simulink model "ControlSystem_Refactorization"  (R2025a)
settings: Solver=FixedStepAuto  StartTime=0.0  StopTime=inf  FixedStep=1e-4  RelTol=1e-3
PostLoadFcn:
  | clear;
  | load_system('ControlSystem_Refactorization');
  | evalin('base', 'run("inicializarBuses.m")');
values from neighbouring files (symbols this model uses):
  actuadorBus = arrayfun(@(x) Simulink.Bus.createMATLABStruct(actuadorBusInfo.busName, x), actuador)    [inicializarBuses.m]
undefined symbols (not defined in the file or in its folder): Configuracion, Controlador, Estado, EstadoValvula, ModoControl, National_Instruments, ParametroControl, PCIe
libraries: simulink x11, sldrtlib x5
(part 1 of 2)
settings Model: SimulationMode=external  ExtModeTrigDuration=10000  Creator=David  LastModifiedBy=David
settings HardwareCC: ProdBitPerLong=64.0  ProdHWDeviceType=Intel->x86-64 (Linux 64)
settings RTWCC: SystemTargetFile=sldrt.tlc  TemplateMakefile=sldrt.tmf  RTWCompilerOptimization=on  Description=Simulink Desktop Real-Time
settings CodeAppCC: MaxIdLength=95.0
settings SimulinkDesktopRealTimeCC: ExtModeTransport=0.0  ExtModeStaticAllocSize=1000000.0  TargetLibSuffix=_sldrt.a  TargetPreCompLibLocation=C:\Program Files\MATLAB\R2025a\toolbox\sldrt\lib\win64  MultiwordLength=2048.0  DynamicStringBufferSize=256.0  ParMdlRefBuildCompliant=on  PreserveMATLABNamespacesInGeneratedCode=on  SubcomponentCodeInterfacePackaging=Reusable function

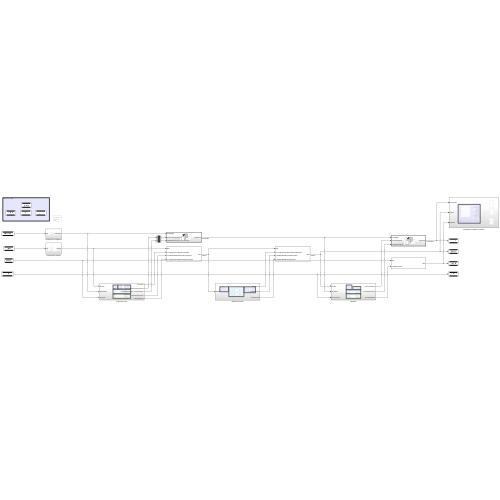
[thumbnail: Simulink's stored preview of the top-level diagram]
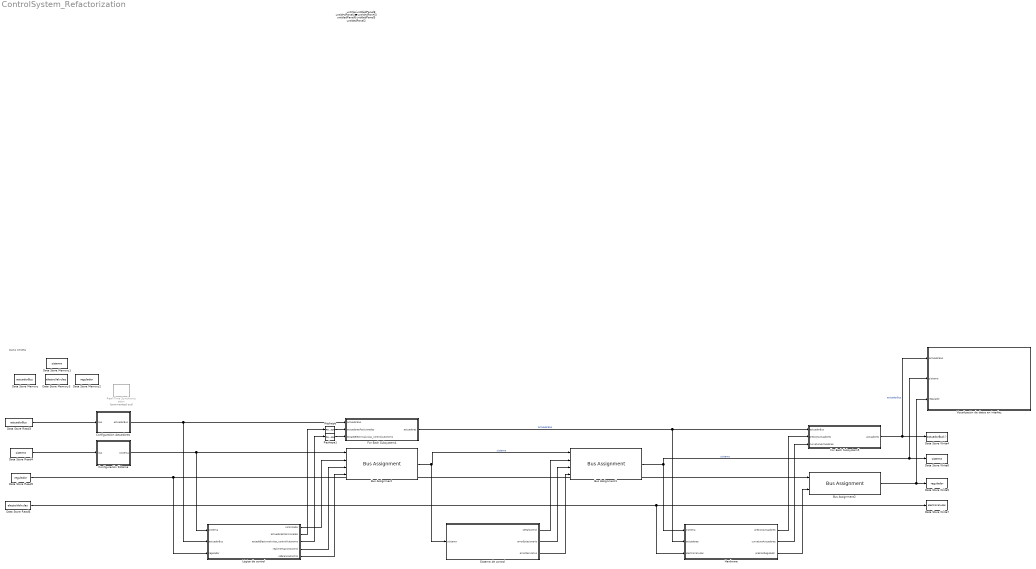
== system ControlSystem_Refactorization ==
  note: DATA STORE
  Bus Assignment : BusAssignment  AssignedSignals=Configuracion.Global.controlador,Estado.Global.realimentacionControl,Configuracion.Global.referenciaControl
  Bus Assignment1 : BusAssignment  AssignedSignals=Configuracion.Global.referenciaControl,Estado.Global.errorEstacionario,Estado.Global.errorDerivativo
  Bus Assignment2 : BusAssignment  AssignedSignals=Estado.presion
  Configuración Actuadores : Subsystem
  Configuración Sistema : Subsystem
  Data Store Memory : DataStoreMemory  DataStoreName=actuadorBus  WriteAfterWriteMsg=warning  InitialValue=actuadorBus  ShowAdditionalParam=off  OutDataTypeStr=Bus: slBusActuador
  Data Store Memory1 : DataStoreMemory  DataStoreName=sistema  WriteAfterWriteMsg=warning  InitialValue=sistema  ShowAdditionalParam=off  OutDataTypeStr=Bus: slBusSistema
  Data Store Memory2 : DataStoreMemory  DataStoreName=regulador  WriteAfterWriteMsg=warning  InitialValue=regulador  ShowAdditionalParam=off  OutDataTypeStr=Bus: slBusRegulador
  Data Store Memory3 : DataStoreMemory  DataStoreName=electroValvulas  WriteAfterWriteMsg=warning  InitialValue=electroValvulas  ShowAdditionalParam=off  OutDataTypeStr=Bus: slBusElectroValvulas
  Data Store Read3 : DataStoreRead  DataStoreName=actuadorBus  IndexOptions=Index vector (dialog)  Indices=1  OutputSizes=1
  Data Store Read4 : DataStoreRead  DataStoreName=sistema  IndexOptions=Index vector (dialog)  Indices=1  OutputSizes=1
  Data Store Read5 : DataStoreRead  DataStoreName=regulador  IndexOptions=Index vector (dialog)  Indices=1  OutputSizes=1
  Data Store Read6 : DataStoreRead  DataStoreName=electroValvulas  IndexOptions=Index vector (dialog)  Indices=1  OutputSizes=1
  Data Store Write4 : DataStoreWrite  DataStoreName=actuadorBus  DataStoreElements=actuadorBus(:)  IndexOptions=Index vector (dialog)  Indices=1  OutputSizes=1
  Data Store Write5 : DataStoreWrite  DataStoreName=regulador  DataStoreElements=regulador  IndexOptions=Index vector (dialog)  Indices=1  OutputSizes=1
  Data Store Write6 : DataStoreWrite  DataStoreName=sistema  DataStoreElements=sistema  IndexOptions=Index vector (dialog)  Indices=1  OutputSizes=1
  Data Store Write7 : DataStoreWrite  DataStoreName=electroValvulas  DataStoreElements=electroValvulas  IndexOptions=Index vector (dialog)  Indices=1  OutputSizes=1
  For Each Subsystem4 : Subsystem  TreatAsAtomicUnit=on
  For Each Subsystem5 : Subsystem  TreatAsAtomicUnit=on
  Hardware : Subsystem
  Lógica de control : Subsystem
  Real-Time Synchronization : sldrtlib/Real-Time Synchronization  Commented=on  SampleTime=0.1  MaxMissedTicks=10  ShowMissedTicks=off  YieldWhenWaiting=off
  Reshape : Reshape  OutputDimensionality=Column vector (2-D)
  Reshape1 : Reshape  OutputDimensionality=Column vector (2-D)
  Sistema de control : Subsystem
  Visualización de datos en interfaz : Subsystem
  untitledPanel : Subsystem  Tag=HiddenForWebPanel  IsWebBlockPanel=on
  untitledPanel1 : Subsystem  Tag=HiddenForWebPanel  IsWebBlockPanel=on
  untitledPanel2 : Subsystem  Tag=HiddenForWebPanel  IsWebBlockPanel=on
  untitledPanel3 : Subsystem  Tag=HiddenForWebPanel  IsWebBlockPanel=on
  untitledPanel4 : Subsystem  Tag=HiddenForWebPanel  IsWebBlockPanel=on
  untitledPanel5 : Subsystem  Tag=HiddenForWebPanel  IsWebBlockPanel=on
  untitledPanel6 : Subsystem  Tag=HiddenForWebPanel  IsWebBlockPanel=on
  untitledPanel8 : Subsystem  Tag=HiddenForWebPanel  IsWebBlockPanel=on
  wires:
  Data Store Read4/1 -> Configuración Sistema/1(bus)
  Data Store Read5/1 -> Lógica de control/3(regulador), Bus Assignment2/1
  Data Store Read3/1 -> Configuración Actuadores/1(bus)
  Lógica de control/1(controlador) -> Bus Assignment/2
  Lógica de control/4(realimentacionControl) -> Bus Assignment/3
  Lógica de control/5(referenciaControl) -> Bus Assignment/4
  Lógica de control/2(actuadoresPosicionados) -> Reshape/1
  Lógica de control/3(estadoElectrovalvulas_controlAutonomo) -> Reshape1/1
  Bus Assignment/1 -> Sistema de control/1(sistema), Bus Assignment1/1  "sistema"
  Sistema de control/1(señalControl) -> Bus Assignment1/2
  Sistema de control/2(errorEstacionario) -> Bus Assignment1/3
  Sistema de control/3(errorDerivativo) -> Bus Assignment1/4
  Bus Assignment1/1 -> Hardware/1(sistema), Visualización de datos en interfaz/2(sistema), Data Store Write6/1  "sistema"
  Data Store Read6/1 -> Data Store Write7/1, Hardware/3(electroValvulas)
  For Each Subsystem4/1(actuadores) -> Hardware/2(actuadores), For Each Subsystem5/1(actuadorBus)  "actuadorBus"
  Hardware/1(presionActuadores) -> For Each Subsystem5/2(presionActuadores)
  Hardware/2(curvaturaActuadores) -> For Each Subsystem5/3(curvaturaActuadores)
  Hardware/3(presiónRegulador) -> Bus Assignment2/2
  For Each Subsystem5/1(actuadores) -> Visualización de datos en interfaz/1(actuadorBus), Data Store Write4/1  "actuadorBus"
  Bus Assignment2/1 -> Visualización de datos en interfaz/3(regulador), Data Store Write5/1
  Reshape/1 -> For Each Subsystem4/2(actuadoresPosicionados)
  Reshape1/1 -> For Each Subsystem4/3(estadoElectrovalvulas_controlAutonomo)
  Configuración Sistema/1(sistema) -> Lógica de control/1(sistema), Bus Assignment/1
  Configuración Actuadores/1(actuadorBus) -> Lógica de control/2(actuadorBus), For Each Subsystem4/1(actuadorBus)

== system ControlSystem_Refactorization/Configuración Actuadores ==
  bus : Inport
  Configuración de usuario : Subsystem  TreatAsAtomicUnit=on
  For Each Subsystem : Subsystem  TreatAsAtomicUnit=on
  actuadorBus : Outport
  wires:
  For Each Subsystem/1(Out1) -> actuadorBus/1
  bus/1 -> For Each Subsystem/1(Bus)
  Configuración de usuario/1(Referencias presión) -> For Each Subsystem/2(Referencias de presión)
  Configuración de usuario/2(Referencias curvatura) -> For Each Subsystem/3(Referencias de curvatura)
  Configuración de usuario/3(Estado válvulas - Control manual) -> For Each Subsystem/4(Estado válvulas - Control manual)
  Configuración de usuario/4(Actuadores activos - Control autónomo) -> For Each Subsystem/5(Actuadores activos - Control autónomo)

== system ControlSystem_Refactorization/Configuración Sistema ==
  bus : Inport
  Bus Assignment3 : BusAssignment  AssignedSignals=Configuracion.Global.modoControl,Configuracion.Global.parametroControl,Configuracion.Global.simulacionActiva,Configuracion.ControlManual.actuadorSeleccionado,Configuracion.Global.ToleranciaPresion.estacionaria,Configuracion.Global.ToleranciaPresion.derivativa,Configuracion.Global.ToleranciaCurvatura.estacionaria,Configuracion.Global.ToleranciaCurvatura.derivativa,Configuracion.Global.toleranciaEquilibrioPresiones
  Configuración de usuario : Subsystem  TreatAsAtomicUnit=on
  sistema : Outport
  wires:
  Bus Assignment3/1 -> sistema/1
  bus/1 -> Bus Assignment3/1
  Configuración de usuario/1(Modo de control) -> Bus Assignment3/2
  Configuración de usuario/2(Parámetro de control) -> Bus Assignment3/3
  Configuración de usuario/3(Simulación activa) -> Bus Assignment3/4
  Configuración de usuario/4(Actuador seleccionado) -> Bus Assignment3/5
  Configuración de usuario/5(Tolerancia Presión Estacionaria) -> Bus Assignment3/6
  Configuración de usuario/6(Tolerancia Presión Derivativa) -> Bus Assignment3/7
  Configuración de usuario/7(Tolerancia Curvatura Estacionaria) -> Bus Assignment3/8
  Configuración de usuario/8(Tolerancia Curvatura Derivativa) -> Bus Assignment3/9
  Configuración de usuario/9(Tolerancia Equilibrio Presiones) -> Bus Assignment3/10

== system ControlSystem_Refactorization/For Each Subsystem4 ==
  actuadorBus : Inport  Partition=on  PartitionDimension=1  PartitionWidth=1  PartitionOffset=0
  actuadoresPosicionados : Inport  Port=2  Partition=on  PartitionDimension=1  PartitionWidth=1  PartitionOffset=0
  estadoElectrovalvulas_controlAutonomo : Inport  Port=3  Partition=on  PartitionDimension=1  PartitionWidth=1  PartitionOffset=0
  Bus Assignment : BusAssignment  AssignedSignals=Estado.ControlAutomatico.actuadorPosicionado,Estado.ControlAutomatico.estadoValvula
  For Each : ForEach  DisableCoverage=on
  actuadores : Outport  ConcatenationDimension=1
  wires:
  actuadorBus/1 -> Bus Assignment/1
  Bus Assignment/1 -> actuadores/1
  actuadoresPosicionados/1 -> Bus Assignment/2
  estadoElectrovalvulas_controlAutonomo/1 -> Bus Assignment/3

== system ControlSystem_Refactorization/For Each Subsystem5 ==
  actuadorBus : Inport  Partition=on  PartitionDimension=1  PartitionWidth=1  PartitionOffset=0
  presionActuadores : Inport  Port=2  Partition=on  PartitionDimension=1  PartitionWidth=1  PartitionOffset=0
  curvaturaActuadores : Inport  Port=3  Partition=on  PartitionDimension=1  PartitionWidth=1  PartitionOffset=0
  Bus Assignment : BusAssignment  AssignedSignals=Estado.Realimentacion.presion,Estado.Realimentacion.curvatura
  For Each : ForEach  DisableCoverage=on
  actuadores : Outport  ConcatenationDimension=1
  wires:
  actuadorBus/1 -> Bus Assignment/1
  Bus Assignment/1 -> actuadores/1
  presionActuadores/1 -> Bus Assignment/2
  curvaturaActuadores/1 -> Bus Assignment/3

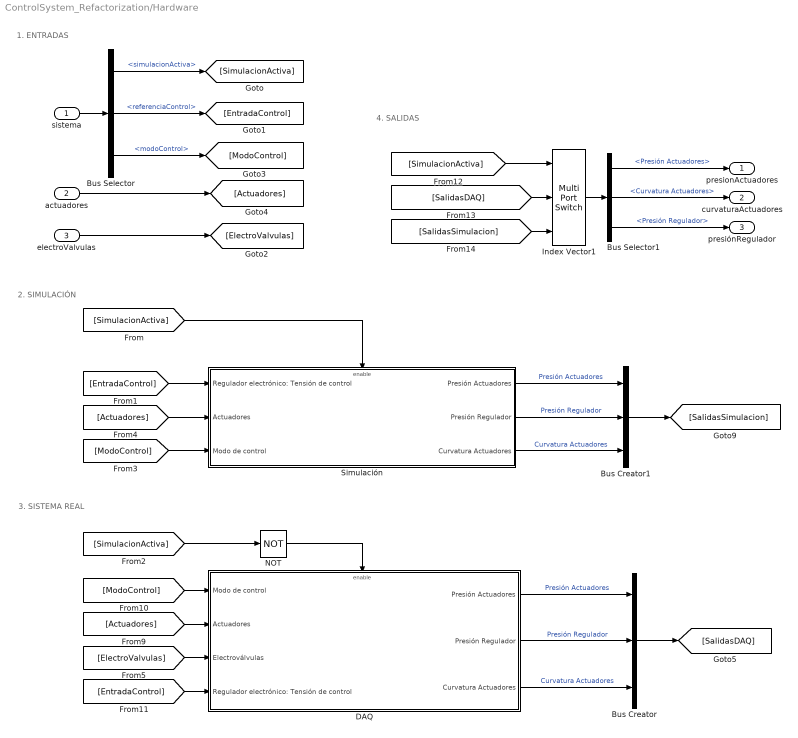
== system ControlSystem_Refactorization/Hardware ==
  note: 3. SISTEMA REAL
  note: 4. SALIDAS
  note: 2. SIMULACIÓN
  note: 1. ENTRADAS
  sistema : Inport
  actuadores : Inport  Port=2
  electroValvulas : Inport  Port=3
  Bus Creator : BusCreator  Inputs=3
  Bus Creator1 : BusCreator  Inputs=3
  Bus Selector : BusSelector  OutputSignals=Configuracion.Global.simulacionActiva,Configuracion.Global.referenciaControl,Configuracion.Global.modoControl
  Bus Selector1 : BusSelector  OutputSignals=Presión Actuadores,Curvatura Actuadores,Presión Regulador
  DAQ : Subsystem  TreatAsAtomicUnit=on
  Index Vector1 : MultiPortSwitch  DataPortOrder=Zero-based contiguous  Inputs=2  DataPortIndices={true,false}  zeroidx=on  SaturateOnIntegerOverflow=off  InputSameDT=off
  NOT : Logic  Operator=NOT  IconShape=distinctive  AllPortsSameDT=off  OutDataTypeStr=boolean
  Simulación : Subsystem  TreatAsAtomicUnit=on
  presionActuadores : Outport
  curvaturaActuadores : Outport  Port=2
  presiónRegulador : Outport  Port=3
  wires:
  sistema/1 -> Bus Selector/1
  Bus Selector/1 -> [SimulacionActiva]  "<simulacionActiva>"
  Bus Selector/2 -> [EntradaControl]  "<referenciaControl>"
  [EntradaControl] -> Simulación/1(Regulador electrónico: Tensión de control)
  [Actuadores] -> Simulación/2(Actuadores)
  Bus Selector/3 -> [ModoControl]  "<modoControl>"
  [ModoControl] -> Simulación/3(Modo de control)
  [SimulacionActiva] -> NOT/1
  electroValvulas/1 -> [ElectroValvulas]
  [ElectroValvulas] -> DAQ/3(Electroválvulas)
  [Actuadores] -> DAQ/2(Actuadores)
  [ModoControl] -> DAQ/1(Modo de control)
  [EntradaControl] -> DAQ/4(Regulador electrónico: Tensión de control)
  DAQ/1(Presión Actuadores) -> Bus Creator/1  "Presión Actuadores"
  NOT/1 -> DAQ/Enable
  [SalidasDAQ] -> Index Vector1/2
  [SalidasSimulacion] -> Index Vector1/3
  [SimulacionActiva] -> Index Vector1/1
  DAQ/3(Curvatura Actuadores) -> Bus Creator/3  "Curvatura Actuadores"
  DAQ/2(Presión Regulador) -> Bus Creator/2  "Presión Regulador"
  Bus Creator/1 -> [SalidasDAQ]
  Simulación/1(Presión Actuadores) -> Bus Creator1/1  "Presión Actuadores"
  Bus Creator1/1 -> [SalidasSimulacion]
  Index Vector1/1 -> Bus Selector1/1
  Bus Selector1/1 -> presionActuadores/1  "<Presión Actuadores>"
  [SimulacionActiva] -> Simulación/Enable
  Simulación/2(Presión Regulador) -> Bus Creator1/2  "Presión Regulador"
  Simulación/3(Curvatura Actuadores) -> Bus Creator1/3  "Curvatura Actuadores"
  Bus Selector1/2 -> curvaturaActuadores/1  "<Curvatura Actuadores>"
  Bus Selector1/3 -> presiónRegulador/1  "<Presión Regulador>"
  actuadores/1 -> [Actuadores]

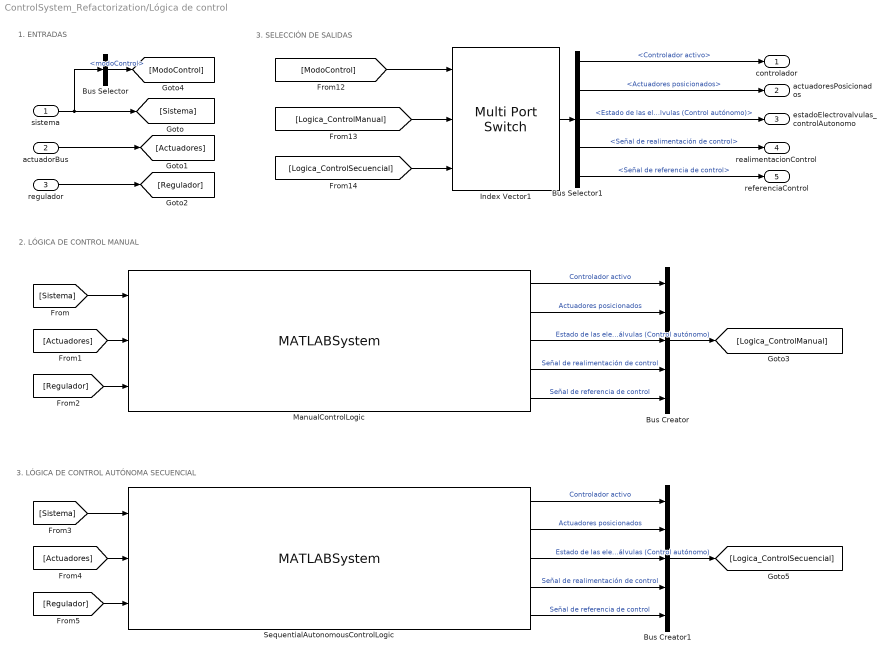
== system ControlSystem_Refactorization/Lógica de control ==
  note: 3. LÓGICA DE CONTROL AUTÓNOMA SECUENCIAL
  note: 3. SELECCIÓN DE SALIDAS
  note: 2. LÓGICA DE CONTROL MANUAL
  note: 1. ENTRADAS
  sistema : Inport
  actuadorBus : Inport  Port=2
  regulador : Inport  Port=3
  Bus Creator : BusCreator  Inputs=5
  Bus Creator1 : BusCreator  Inputs=5
  Bus Selector : BusSelector  OutputSignals=Configuracion.Global.modoControl
  Bus Selector1 : BusSelector  OutputSignals=|
      | Controlador activo,Actuadores posicionados,Estado de las electroválvulas
      | (Control autónomo),Señal de realimentación de control,Señal de referencia de control
  Index Vector1 : MultiPortSwitch  DataPortOrder=Specify indices  Inputs=2  DataPortIndices={ModoControl.Manual,ModoControl.Autonomo_Secuencial}  SaturateOnIntegerOverflow=off  InputSameDT=off
  ManualControlLogic : MATLABSystem  System=manualControlLogic  SimulateUsing=Code generation
      mask Type: manualControlLogic
  SequentialAutonomousControlLogic : MATLABSystem  System=sequential_autonomousControlLogic  numAct=numAct  SimulateUsing=Code generation
      mask Type: sequential_autonomousControlLogic
  controlador : Outport
  actuadoresPosicionados : Outport  Port=2
  estadoElectrovalvulas_controlAutonomo : Outport  Port=3
  realimentacionControl : Outport  Port=4
  referenciaControl : Outport  Port=5
  wires:
  sistema/1 -> Bus Selector/1, [Sistema]
  [Sistema] -> ManualControlLogic/1
  actuadorBus/1 -> [Actuadores]
  regulador/1 -> [Regulador]
  [Regulador] -> ManualControlLogic/3
  [Actuadores] -> ManualControlLogic/2
  ManualControlLogic/1 -> Bus Creator/1  "Controlador activo"
  ManualControlLogic/2 -> Bus Creator/2  "Actuadores posicionados"
  ManualControlLogic/3 -> Bus Creator/3  "Estado de las electroválvulas (Control autónomo)"
  ManualControlLogic/4 -> Bus Creator/4  "Señal de realimentación de control"
  ManualControlLogic/5 -> Bus Creator/5  "Señal de referencia de control"
  Bus Creator/1 -> [Logica_ControlManual]
  [ModoControl] -> Index Vector1/1
  [Logica_ControlSecuencial] -> Index Vector1/3
  Index Vector1/1 -> Bus Selector1/1
  [Logica_ControlManual] -> Index Vector1/2
  Bus Selector/1 -> [ModoControl]  "<modoControl>"
  Bus Selector1/1 -> controlador/1  "<Controlador activo>"
  Bus Selector1/2 -> actuadoresPosicionados/1  "<Actuadores posicionados>"
  Bus Selector1/3 -> estadoElectrovalvulas_controlAutonomo/1  "<Estado de las electroválvulas (Control autónomo)>"
  Bus Selector1/4 -> realimentacionControl/1  "<Señal de realimentación de control>"
  Bus Selector1/5 -> referenciaControl/1  "<Señal de referencia de control>"
  [Sistema] -> SequentialAutonomousControlLogic/1
  [Regulador] -> SequentialAutonomousControlLogic/3
  [Actuadores] -> SequentialAutonomousControlLogic/2
  SequentialAutonomousControlLogic/2 -> Bus Creator1/2  "Actuadores posicionados"
  SequentialAutonomousControlLogic/1 -> Bus Creator1/1  "Controlador activo"
  SequentialAutonomousControlLogic/5 -> Bus Creator1/5  "Señal de referencia de control"
  SequentialAutonomousControlLogic/3 -> Bus Creator1/3  "Estado de las electroválvulas (Control autónomo)"
  Bus Creator1/1 -> [Logica_ControlSecuencial]
  SequentialAutonomousControlLogic/4 -> Bus Creator1/4  "Señal de realimentación de control"

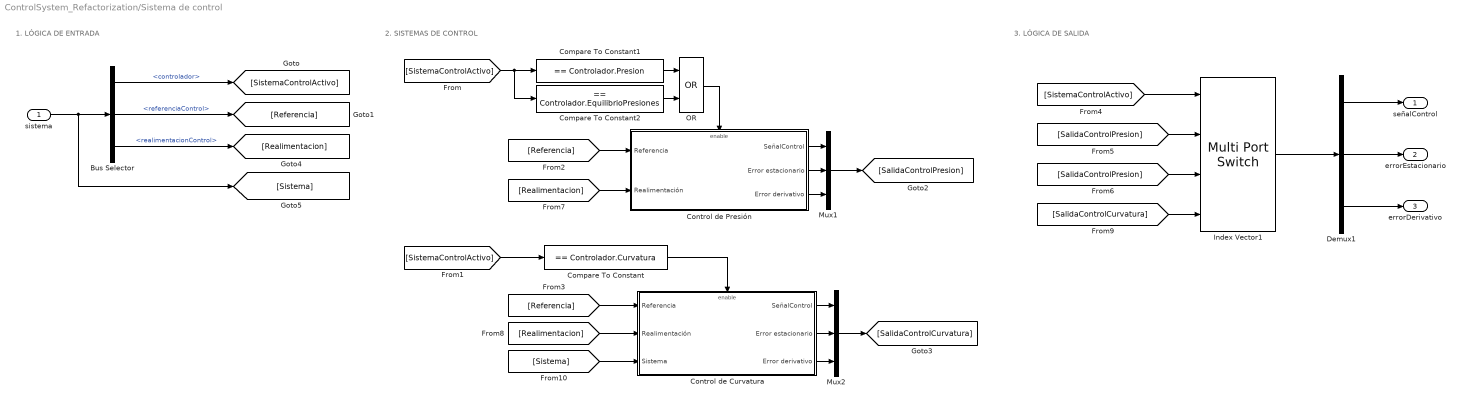
== system ControlSystem_Refactorization/Sistema de control ==
  note: 3. LÓGICA DE SALIDA
  note: 2. SISTEMAS DE CONTROL
  note: 1. LÓGICA DE ENTRADA
  sistema : Inport
  Bus Selector : BusSelector  OutputSignals=Configuracion.Global.controlador,Configuracion.Global.referenciaControl,Estado.Global.realimentacionControl
  Compare To Constant : simulink/Logic and Bit Operations/Compare To Constant  relop===  const=Controlador.Curvatura  OutDataTypeStr=boolean
  Compare To Constant1 : simulink/Logic and Bit Operations/Compare To Constant  relop===  const=Controlador.Presion  OutDataTypeStr=boolean
  Compare To Constant2 : simulink/Logic and Bit Operations/Compare To Constant  relop===  const=Controlador.EquilibrioPresiones  OutDataTypeStr=boolean
  Control de Curvatura : Subsystem  TreatAsAtomicUnit=on  VariantControl=sistemaControlActivo == 0
  Control de Presión : Subsystem  TreatAsAtomicUnit=on  VariantControl=sistemaControlActivo == 1
  Demux1 : Demux  Outputs=3
  Index Vector1 : MultiPortSwitch  DataPortOrder=Specify indices  Inputs=2  DataPortIndices={Controlador.Presion,Controlador.EquilibrioPresiones,Controlador.Curvatura}  SaturateOnIntegerOverflow=off  InputSameDT=off
  Mux1 : Mux  Inputs=3
  Mux2 : Mux  Inputs=3
  OR : Logic  Operator=OR  AllPortsSameDT=off  OutDataTypeStr=boolean
  señalControl : Outport
  errorEstacionario : Outport  Port=2
  errorDerivativo : Outport  Port=3
  wires:
  Bus Selector/2 -> [Referencia]  "<referenciaControl>"
  sistema/1 -> [Sistema], Bus Selector/1
  Bus Selector/3 -> [Realimentacion]  "<realimentacionControl>"
  Compare To Constant/1 -> Control de Curvatura/Enable
  [SistemaControlActivo] -> Compare To Constant1/1, Compare To Constant2/1
  [SistemaControlActivo] -> Compare To Constant/1
  [Referencia] -> Control de Presión/1(Referencia)
  [Realimentacion] -> Control de Presión/2(Realimentación)
  Control de Presión/1(SeñalControl) -> Mux1/1
  Control de Presión/2(Error estacionario) -> Mux1/2
  Control de Presión/3(Error derivativo) -> Mux1/3
  Index Vector1/1 -> Demux1/1
  Demux1/1 -> señalControl/1
  Demux1/2 -> errorEstacionario/1
  Demux1/3 -> errorDerivativo/1
  Control de Curvatura/3(Error derivativo) -> Mux2/3
  Control de Curvatura/2(Error estacionario) -> Mux2/2
  [SistemaControlActivo] -> Index Vector1/1
  Mux1/1 -> [SalidaControlPresion]
  Mux2/1 -> [SalidaControlCurvatura]
  [SalidaControlPresion] -> Index Vector1/2
  [SalidaControlPresion] -> Index Vector1/3
  Control de Curvatura/1(SeñalControl) -> Mux2/1
  Bus Selector/1 -> [SistemaControlActivo]  "<controlador>"
  Compare To Constant1/1 -> OR/1
  Compare To Constant2/1 -> OR/2
  OR/1 -> Control de Presión/Enable
  [Referencia] -> Control de Curvatura/1(Referencia)
  [Realimentacion] -> Control de Curvatura/2(Realimentación)
  [SalidaControlCurvatura] -> Index Vector1/4
  [Sistema] -> Control de Curvatura/3(Sistema)

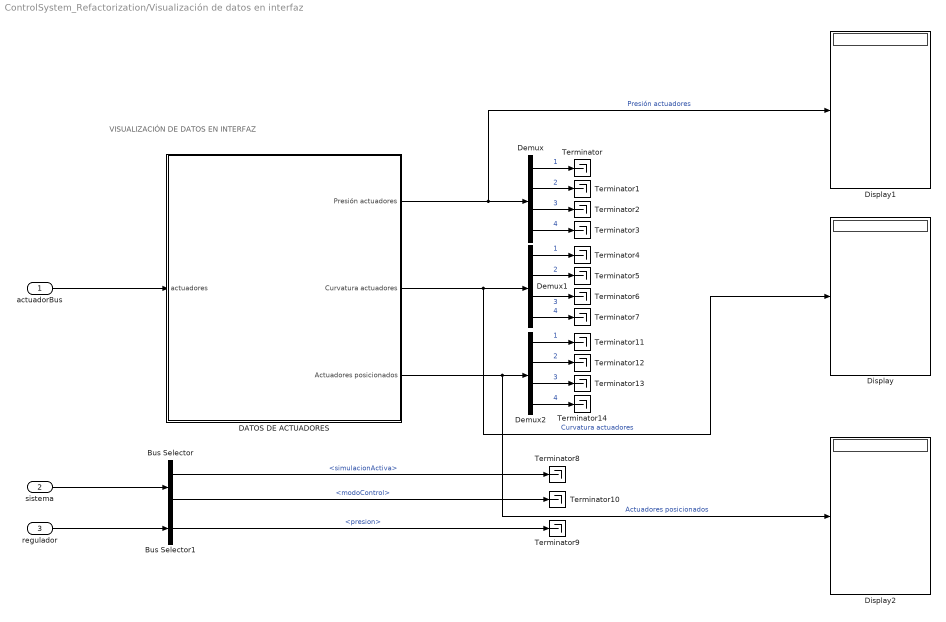
== system ControlSystem_Refactorization/Visualización de datos en interfaz ==
  note: VISUALIZACIÓN DE DATOS EN INTERFAZ
  actuadorBus : Inport
  sistema : Inport  Port=2
  regulador : Inport  Port=3
  Bus Selector : BusSelector  OutputSignals=Configuracion.Global.simulacionActiva,Configuracion.Global.modoControl
  Bus Selector1 : BusSelector  OutputSignals=Estado.presion
  DATOS DE ACTUADORES : Subsystem  TreatAsAtomicUnit=on
  Demux : Demux
  Demux1 : Demux
  Demux2 : Demux
  Display : Display
  Display1 : Display
  Display2 : Display
  Terminator{,1..14} (15 alike) : Terminator
  wires:
  DATOS DE ACTUADORES/3(Actuadores posicionados) -> Display2/1, Demux2/1  "Actuadores posicionados"
  Bus Selector/2 -> Terminator10/1  "<modoControl>"
  Demux1/2 -> Terminator5/1  "2"
  Bus Selector/1 -> Terminator8/1  "<simulacionActiva>"
  Demux1/3 -> Terminator6/1  "3"
  Demux/2 -> Terminator1/1  "2"
  sistema/1 -> Bus Selector/1
  Demux2/2 -> Terminator12/1  "2"
  Demux2/1 -> Terminator11/1  "1"
  Demux/1 -> Terminator/1  "1"
  Demux2/4 -> Terminator14/1  "4"
  Bus Selector1/1 -> Terminator9/1  "<presion>"
  Demux1/4 -> Terminator7/1  "4"
  Demux2/3 -> Terminator13/1  "3"
  Demux/3 -> Terminator2/1  "3"
  DATOS DE ACTUADORES/2(Curvatura actuadores) -> Display/1, Demux1/1  "Curvatura actuadores"
  Demux1/1 -> Terminator4/1  "1"
  Demux/4 -> Terminator3/1  "4"
  actuadorBus/1 -> DATOS DE ACTUADORES/1(actuadores)
  DATOS DE ACTUADORES/1(Presión actuadores) -> Display1/1, Demux/1  "Presión actuadores"
  regulador/1 -> Bus Selector1/1

== system ControlSystem_Refactorization/untitledPanel ==
  Radio Button : RadioButtonGroup  Tag=HiddenForWebPanel  PanelInfo="{\"height\":100,\"left\":11,\"panelId\":\"panelId-fb0ad488-5db8-42e2-ae0e-253fdd9a5e68\",\"top\":40,\"type\":\"panelChild\",\"version\":\"2019b\",\"width\":132,\"zIndex\":1500006}"  LabelPosition=Hide  SelectedLabel=Presion  ButtonGroupName=Parámetro de Control  UseEnumeratedDataType=on  EnumeratedDataType=ParametroControl
  Radio Button1 : RadioButtonGroup  Tag=HiddenForWebPanel  PanelInfo="{\"height\":99,\"left\":145,\"panelId\":\"panelId-fb0ad488-5db8-42e2-ae0e-253fdd9a5e68\",\"top\":42,\"type\":\"panelChild\",\"version\":\"2019b\",\"width\":143,\"zIndex\":1500004}"  LabelPosition=Hide  SelectedLabel=Autonomo_Secuencial  ButtonGroupName=Modo de Control  UseEnumeratedDataType=on  EnumeratedDataType=ModoControl
  panelInfo : PanelWebBlock  Tag=HiddenForWebPanel  PanelInfo="{\"compacted\":false,\"height\":151,\"isActiveTab\":true,\"labels\":{\"label2392456915\":{\"deleted\":false,\"left\":62,\"settings\":{\"backgroundColor\":\"rgba(0, 0, 0, 0)\",\"bold\":true,\"font\":\"Arial\",\"fontColor\":\"black\",\"fontSize\":0.93,\"italicized\":false,\"underlined\":false},\"text\":\"SISTEMA DE CONTROL\",\"top\":11}},\"left\":15,\"name\":\"Sistema de Control\",\"panelId\":\"panelId-fb0ad488-5db8-42e2-ae0e-253fdd9a5e68\",\"tabIndex\":0,\"tabbedSetId\":\"tabbedSet9951176802\",\"top\":26,\"type\":\"panel\",\"version\":\"2019b\",\"visible\":true,\"width\":302,\"zIndex\":1499998}"  PanelSnapshot=<binary blob, 19984 chars, not shown>

== system ControlSystem_Refactorization/untitledPanel1 ==
  Slider : SliderBlock  Tag=HiddenForWebPanel  PanelInfo="{\"height\":91,\"left\":18,\"panelId\":\"panelId-0a77c4da-c2a8-41ad-8fe5-810be4e28cdd\",\"top\":60,\"type\":\"panelChild\",\"version\":\"2019b\",\"width\":408,\"zIndex\":1500002}"  LabelPosition=Hide  ScaleMax=1  TickInterval=0.2
  Slider1 : SliderBlock  Tag=HiddenForWebPanel  PanelInfo="{\"height\":91,\"left\":20,\"panelId\":\"panelId-0a77c4da-c2a8-41ad-8fe5-810be4e28cdd\",\"top\":186,\"type\":\"panelChild\",\"version\":\"2019b\",\"width\":401,\"zIndex\":1500004}"  LabelPosition=Hide  ScaleMax=1  TickInterval=0.2
  Slider2 : SliderBlock  Tag=HiddenForWebPanel  PanelInfo="{\"height\":94,\"left\":20,\"panelId\":\"panelId-0a77c4da-c2a8-41ad-8fe5-810be4e28cdd\",\"top\":316,\"type\":\"panelChild\",\"version\":\"2019b\",\"width\":397,\"zIndex\":1500006}"  LabelPosition=Hide  ScaleMax=1  TickInterval=0.2
  Slider3 : SliderBlock  Tag=HiddenForWebPanel  PanelInfo="{\"height\":98,\"left\":16,\"panelId\":\"panelId-0a77c4da-c2a8-41ad-8fe5-810be4e28cdd\",\"top\":453,\"type\":\"panelChild\",\"version\":\"2019b\",\"width\":400,\"zIndex\":1500008}"  LabelPosition=Hide  ScaleMax=1  TickInterval=0.2
  panelInfo : PanelWebBlock  Tag=HiddenForWebPanel  PanelInfo="{\"compacted\":false,\"height\":591,\"isActiveTab\":true,\"labels\":{\"label0092200108\":{\"deleted\":false,\"left\":188,\"settings\":{\"backgroundColor\":\"rgba(0, 0, 0, 0)\",\"bold\":false,\"font\":\"Arial\",\"fontColor\":\"black\",\"fontSize\":0.93,\"italicized\":false,\"underlined\":false},\"text\":\"Actuador 1\",\"top\":152},\"label1153225224\":{\"deleted\":false,\"left\":181,\"settings\":{\"backgroundColor\":\"rgba(0, 0, 0, 0)\",\"bold\":false,\"font\":\"Arial\",\"fontColor\":\"black\",\"fontSize\":0.93,\"italicized\":false,\"underlined\":false},\"text\":\"Actuador 2\",\"top\":283},\"label1314078370\":{\"deleted\":false,\"left\":180,\"settings\":{\"backgroundColor\":\"rgba(0, 0, 0, 0)\",\"bold\":false,\"font\":\"Arial\",\"fontColor\":\"black\",\"fontSize\":0.93,\"italicized\":false,\"underlined\":false},\"text\":\"Actuador 3\",\"top\":411},\"label3420356265\":{\"deleted\":false,\"left\":181,\"settings\":{\"backgroundColor\":\"rgba(0, 0, 0, 0)\",\"bold\":false,\"font\":\"Arial\",\"fontColor\":\"black\",\"fontSize\":0.93,\"italicized\":false,\"underlined\":false},\"text\":\"Actuador 4\",\"top\":553},\"label3683283443\":{\"deleted\":false,\"left\":99,\"settings\":{\"backgroundColor\":\"rgba(0, 0, 0, 0)\",\"bold\":true,\"font\":\"Arial\",\"fontColor\":\"black\",\"fontSize\":1.03,\"italicized\":false,\"underlined\":false},\"text\":\"REFERENCIAS DE CONTROL\",\"top\":10},\"label7967686149\":{\"deleted\":false,\"left\":190,\"settings\":{\"backgroundColor\":\"rgba(0, 0, 0, 0)\",\"bold\":true,\"font\":\"Arial\",\"fontColor\":\"black\",\"fontSize\":0.93,\"italicized\":false,\"underlined\":false},\"text\":\"PRESIÓN\",\"top\":38}},\"left\":19,\"name\":\"Referencias: Presión\",\"panelId\":\"panelId-0a77c4da-c2a8-41ad-8fe5-810be4e28cdd\",\"tabIndex\":0,\"tabbedSetId\":\"tabbedSet7116138444\",\"top\":202,\"type\":\"panel\",\"version\":\"2019b\",\"visible\":true,\"width\":436,\"zIndex\":1500002}"  PanelSnapshot=<binary blob, 44904 chars, not shown>

== system ControlSystem_Refactorization/untitledPanel2 ==
  Slider : SliderBlock  Tag=HiddenForWebPanel  PanelInfo="{\"height\":101,\"left\":16,\"panelId\":\"panelId-efc9d301-ffcb-4978-afbf-6fdea22ede6f\",\"top\":64,\"type\":\"panelChild\",\"version\":\"2019b\",\"width\":401,\"zIndex\":1500002}"  LabelPosition=Hide  ScaleMax=0.024  TickInterval=0.004
  Slider1 : SliderBlock  Tag=HiddenForWebPanel  PanelInfo="{\"height\":89,\"left\":19,\"panelId\":\"panelId-efc9d301-ffcb-4978-afbf-6fdea22ede6f\",\"top\":198,\"type\":\"panelChild\",\"version\":\"2019b\",\"width\":395,\"zIndex\":1500004}"  LabelPosition=Hide  ScaleMax=0.024  TickInterval=0.004
  Slider2 : SliderBlock  Tag=HiddenForWebPanel  PanelInfo="{\"height\":94,\"left\":20,\"panelId\":\"panelId-efc9d301-ffcb-4978-afbf-6fdea22ede6f\",\"top\":323,\"type\":\"panelChild\",\"version\":\"2019b\",\"width\":391,\"zIndex\":1500006}"  LabelPosition=Hide  ScaleMax=0.024  TickInterval=0.004
  Slider3 : SliderBlock  Tag=HiddenForWebPanel  PanelInfo="{\"height\":100,\"left\":23,\"panelId\":\"panelId-efc9d301-ffcb-4978-afbf-6fdea22ede6f\",\"top\":453,\"type\":\"panelChild\",\"version\":\"2019b\",\"width\":384,\"zIndex\":1500008}"  LabelPosition=Hide  ScaleMax=0.024  TickInterval=0.004
  panelInfo : PanelWebBlock  Tag=HiddenForWebPanel  PanelInfo="{\"compacted\":false,\"height\":594,\"isActiveTab\":false,\"labels\":{\"label0573807186\":{\"deleted\":false,\"left\":175,\"settings\":{\"backgroundColor\":\"rgba(0, 0, 0, 0)\",\"bold\":false,\"font\":\"Arial\",\"fontColor\":\"black\",\"fontSize\":0.9,\"italicized\":false,\"underlined\":false},\"text\":\"Actuador 3\",\"top\":419},\"label1621129159\":{\"deleted\":false,\"left\":173,\"settings\":{\"backgroundColor\":\"rgba(0, 0, 0, 0)\",\"bold\":false,\"font\":\"Arial\",\"fontColor\":\"black\",\"fontSize\":0.9,\"italicized\":false,\"underlined\":false},\"text\":\"Actuador 4\",\"top\":556},\"label4453390890\":{\"deleted\":false,\"left\":176,\"settings\":{\"backgroundColor\":\"rgba(0, 0, 0, 0)\",\"bold\":false,\"font\":\"Arial\",\"fontColor\":\"black\",\"fontSize\":0.9,\"italicized\":false,\"underlined\":false},\"text\":\"Actuador 2\",\"top\":289},\"label7755809631\":{\"deleted\":false,\"left\":179,\"settings\":{\"backgroundColor\":\"rgba(0, 0, 0, 0)\",\"bold\":false,\"font\":\"Arial\",\"fontColor\":\"black\",\"fontSize\":0.9,\"italicized\":false,\"underlined\":false},\"text\":\"Actuador 1\",\"top\":167},\"label7970316676\":{\"deleted\":false,\"left\":164,\"settings\":{\"backgroundColor\":\"rgba(0, 0, 0, 0)\",\"bold\":true,\"font\":\"Arial\",\"fontColor\":\"black\",\"fontSize\":1,\"italicized\":false,\"underlined\":false},\"text\":\"CURVATURA\",\"top\":39},\"label9571937969\":{\"deleted\":false,\"left\":89,\"settings\":{\"backgroundColor\":\"rgba(0, 0, 0, 0)\",\"bold\":true,\"font\":\"Arial\",\"fontColor\":\"black\",\"fontSize\":1.1,\"italicized\":false,\"underlined\":false},\"text\":\"REFERENCIAS DE CONTROL\",\"top\":12}},\"left\":19,\"name\":\"Referencias: Curvatura\",\"panelId\":\"panelId-efc9d301-ffcb-4978-afbf-6fdea22ede6f\",\"tabIndex\":1,\"tabbedSetId\":\"tabbedSet7116138444\",\"top\":202,\"type\":\"panel\",\"version\":\"2019b\",\"visible\":false,\"width\":433,\"zIndex\":1500004}"  PanelSnapshot=<binary blob, 50268 chars, not shown>

== system ControlSystem_Refactorization/untitledPanel3 ==
  Linear Gauge : LinearGaugeBlock  Tag=HiddenForWebPanel  PanelInfo="{\"height\":89,\"left\":11,\"panelId\":\"panelId-822440f7-b699-41c8-b6b7-d3232cbf51ea\",\"top\":243,\"type\":\"panelChild\",\"version\":\"2019b\",\"width\":375,\"zIndex\":1500008}"  LabelPosition=Hide  ScaleMax=1  TickInterval=0.1  FontColor=[0.0, 0.0, 0.0]
  Linear Gauge1 : LinearGaugeBlock  Tag=HiddenForWebPanel  PanelInfo="{\"height\":84,\"left\":10,\"panelId\":\"panelId-822440f7-b699-41c8-b6b7-d3232cbf51ea\",\"top\":371,\"type\":\"panelChild\",\"version\":\"2019b\",\"width\":376,\"zIndex\":1500004}"  LabelPosition=Hide  ScaleMax=1  TickInterval=0.1  FontColor=[0.0, 0.0, 0.0]
  Linear Gauge2 : LinearGaugeBlock  Tag=HiddenForWebPanel  PanelInfo="{\"height\":81,\"left\":12,\"panelId\":\"panelId-822440f7-b699-41c8-b6b7-d3232cbf51ea\",\"top\":498,\"type\":\"panelChild\",\"version\":\"2019b\",\"width\":376,\"zIndex\":1500006}"  LabelPosition=Hide  ScaleMax=1  TickInterval=0.1  FontColor=[0.0, 0.0, 0.0]
  Linear Gauge3 : LinearGaugeBlock  Tag=HiddenForWebPanel  PanelInfo="{\"height\":85,\"left\":12,\"panelId\":\"panelId-822440f7-b699-41c8-b6b7-d3232cbf51ea\",\"top\":624,\"type\":\"panelChild\",\"version\":\"2019b\",\"width\":377,\"zIndex\":1500002}"  LabelPosition=Hide  ScaleMax=1  TickInterval=0.1  FontColor=[0.0, 0.0, 0.0]
  Linear Gauge4 : LinearGaugeBlock  Tag=HiddenForWebPanel  PanelInfo="{\"height\":81,\"left\":13,\"panelId\":\"panelId-822440f7-b699-41c8-b6b7-d3232cbf51ea\",\"top\":76,\"type\":\"panelChild\",\"version\":\"2019b\",\"width\":371,\"zIndex\":1500010}"  LabelPosition=Hide  ScaleMax=1  TickInterval=0.1  FontColor=[0.0, 0.0, 0.0]
  panelInfo : PanelWebBlock  Tag=HiddenForWebPanel  PanelInfo="{\"compacted\":false,\"height\":769,\"isActiveTab\":true,\"labels\":{\"label0385178640\":{\"deleted\":false,\"left\":75,\"settings\":{\"backgroundColor\":\"rgba(0, 0, 0, 0)\",\"bold\":true,\"font\":\"Arial\",\"fontColor\":\"black\",\"fontSize\":0.95,\"italicized\":false,\"underlined\":false},\"text\":\"REALIMENTACIÓN DEL REGULADOR\",\"top\":16},\"label1724135462\":{\"deleted\":false,\"left\":163,\"settings\":{\"backgroundColor\":\"rgba(0, 0, 0, 0)\",\"bold\":false,\"font\":\"Arial\",\"fontColor\":\"black\",\"fontSize\":0.95,\"italicized\":false,\"underlined\":false},\"text\":\"Actuador 3\",\"top\":583},\"label2150277251\":{\"deleted\":false,\"left\":167,\"settings\":{\"backgroundColor\":\"rgba(0, 0, 0, 0)\",\"bold\":false,\"font\":\"Arial\",\"fontColor\":\"black\",\"fontSize\":0.95,\"italicized\":false,\"underlined\":false},\"text\":\"Actuador 2\",\"top\":460},\"label3680534337\":{\"deleted\":false,\"left\":162,\"settings\":{\"backgroundColor\":\"rgba(0, 0, 0, 0)\",\"bold\":false,\"font\":\"Arial\",\"fontColor\":\"black\",\"fontSize\":0.95,\"italicized\":false,\"underlined\":false},\"text\":\"Actuador 4\",\"top\":714},\"label6954658628\":{\"deleted\":false,\"left\":167,\"settings\":{\"backgroundColor\":\"rgba(0, 0, 0, 0)\",\"bold\":false,\"font\":\"Arial\",\"fontColor\":\"black\",\"fontSize\":0.95,\"italicized\":false,\"underlined\":false},\"text\":\"Actuador 1\",\"top\":338},\"label7110062360\":{\"deleted\":false,\"left\":74,\"settings\":{\"backgroundColor\":\"rgba(0, 0, 0, 0)\",\"bold\":true,\"font\":\"Arial\",\"fontColor\":\"black\",\"fontSize\":1.06,\"italicized\":false,\"underlined\":false},\"text\":\"REALIMENTACIÓN DE CONTROL\",\"top\":189},\"label7831479186\":{\"deleted\":false,\"left\":170,\"settings\":{\"backgroundColor\":\"rgba(0, 0, 0, 0)\",\"bold\":true,\"font\":\"Arial\",\"fontColor\":\"black\",\"fontSize\":0.85,\"italicized\":false,\"underlined\":false},\"text\":\"PRESIÓN\",\"top\":43},\"label9355264038\":{\"deleted\":false,\"left\":168,\"settings\":{\"backgroundColor\":\"rgba(0, 0, 0, 0)\",\"bold\":true,\"font\":\"Arial\",\"fontColor\":\"black\",\"fontSize\":0.95,\"italicized\":false,\"underlined\":false},\"text\":\"PRESIÓN\",\"top\":219}},\"left\":455,\"name\":\"Realimentación - Presión\",\"panelId\":\"panelId-822440f7-b699-41c8-b6b7-d3232cbf51ea\",\"tabIndex\":0,\"tabbedSetId\":\"tabbedSet0999669587\",\"top\":25,\"type\":\"panel\",\"version\":\"2019b\",\"visible\":true,\"width\":397,\"zIndex\":1500006}"  PanelSnapshot=<binary blob, 71116 chars, not shown>

== system ControlSystem_Refactorization/untitledPanel4 ==
  Edit : EditField  Tag=HiddenForWebPanel  PanelInfo="{\"height\":25,\"left\":19,\"panelId\":\"panelId-e9df1c98-1b0a-4be2-b494-28bc6a7653a3\",\"top\":234,\"type\":\"panelChild\",\"version\":\"2019b\",\"width\":99,\"zIndex\":1500018}"  LabelPosition=Hide  ShowInitialText=on  Alignment=Center
  Edit1 : EditField  Tag=HiddenForWebPanel  PanelInfo="{\"height\":27,\"left\":137,\"panelId\":\"panelId-e9df1c98-1b0a-4be2-b494-28bc6a7653a3\",\"top\":234,\"type\":\"panelChild\",\"version\":\"2019b\",\"width\":92,\"zIndex\":1500020}"  LabelPosition=Hide  ShowInitialText=on  Alignment=Center
  Edit2 : EditField  Tag=HiddenForWebPanel  PanelInfo="{\"height\":26,\"left\":18,\"panelId\":\"panelId-e9df1c98-1b0a-4be2-b494-28bc6a7653a3\",\"top\":283,\"type\":\"panelChild\",\"version\":\"2019b\",\"width\":100,\"zIndex\":1500030}"  LabelPosition=Hide  ShowInitialText=on  Alignment=Center
  Edit3 : EditField  Tag=HiddenForWebPanel  PanelInfo="{\"height\":29,\"left\":138,\"panelId\":\"panelId-e9df1c98-1b0a-4be2-b494-28bc6a7653a3\",\"top\":285,\"type\":\"panelChild\",\"version\":\"2019b\",\"width\":90,\"zIndex\":1500032}"  LabelPosition=Hide  ShowInitialText=on  Alignment=Center
  Edit4 : EditField  Tag=HiddenForWebPanel  PanelInfo="{\"height\":29,\"left\":254,\"panelId\":\"panelId-e9df1c98-1b0a-4be2-b494-28bc6a7653a3\",\"top\":231,\"type\":\"panelChild\",\"version\":\"2019b\",\"width\":89,\"zIndex\":1500034}"  LabelPosition=Hide  ShowInitialText=on  Alignment=Center
  Lamp : LampBlock  Tag=HiddenForWebPanel  PanelInfo="{\"height\":105,\"left\":42,\"panelId\":\"panelId-e9df1c98-1b0a-4be2-b494-28bc6a7653a3\",\"top\":372,\"type\":\"panelChild\",\"version\":\"2019b\",\"width\":114,\"zIndex\":1500002}"  LabelPosition=Hide  DefaultColor=[192.0, 192.0, 192.0]
  Lamp1 : LampBlock  Tag=HiddenForWebPanel  PanelInfo="{\"height\":105,\"left\":214,\"panelId\":\"panelId-e9df1c98-1b0a-4be2-b494-28bc6a7653a3\",\"top\":375,\"type\":\"panelChild\",\"version\":\"2019b\",\"width\":114,\"zIndex\":1500004}"  LabelPosition=Hide  DefaultColor=[192.0, 192.0, 192.0]
  Lamp2 : LampBlock  Tag=HiddenForWebPanel  PanelInfo="{\"height\":105,\"left\":43,\"panelId\":\"panelId-e9df1c98-1b0a-4be2-b494-28bc6a7653a3\",\"top\":566,\"type\":\"panelChild\",\"version\":\"2019b\",\"width\":114,\"zIndex\":1500006}"  LabelPosition=Hide  DefaultColor=[192.0, 192.0, 192.0]
  Lamp3 : LampBlock  Tag=HiddenForWebPanel  PanelInfo="{\"height\":105,\"left\":218,\"panelId\":\"panelId-e9df1c98-1b0a-4be2-b494-28bc6a7653a3\",\"top\":568,\"type\":\"panelChild\",\"version\":\"2019b\",\"width\":114,\"zIndex\":1500008}"  LabelPosition=Hide  DefaultColor=[192.0, 192.0, 192.0]
  Lamp4 : LampBlock  Tag=HiddenForWebPanel  PanelInfo="{\"height\":105,\"left\":126,\"panelId\":\"panelId-e9df1c98-1b0a-4be2-b494-28bc6a7653a3\",\"top\":50,\"type\":\"panelChild\",\"version\":\"2019b\",\"width\":114,\"zIndex\":1500022}"  LabelPosition=Hide  DefaultColor=[192.0, 192.0, 192.0]
  Slider Switch1 : SliderSwitchBlock  Tag=HiddenForWebPanel  PanelInfo="{\"height\":46,\"left\":44,\"panelId\":\"panelId-e9df1c98-1b0a-4be2-b494-28bc6a7653a3\",\"top\":485,\"type\":\"panelChild\",\"version\":\"2019b\",\"width\":114,\"zIndex\":1500010}"  LabelPosition=Hide
  Slider Switch2 : SliderSwitchBlock  Tag=HiddenForWebPanel  PanelInfo="{\"height\":45,\"left\":212,\"panelId\":\"panelId-e9df1c98-1b0a-4be2-b494-28bc6a7653a3\",\"top\":489,\"type\":\"panelChild\",\"version\":\"2019b\",\"width\":121,\"zIndex\":1500012}"  LabelPosition=Hide
  Slider Switch3 : SliderSwitchBlock  Tag=HiddenForWebPanel  PanelInfo="{\"height\":45,\"left\":48,\"panelId\":\"panelId-e9df1c98-1b0a-4be2-b494-28bc6a7653a3\",\"top\":677,\"type\":\"panelChild\",\"version\":\"2019b\",\"width\":110,\"zIndex\":1500014}"  LabelPosition=Hide
  Slider Switch4 : SliderSwitchBlock  Tag=HiddenForWebPanel  PanelInfo="{\"height\":44,\"left\":220,\"panelId\":\"panelId-e9df1c98-1b0a-4be2-b494-28bc6a7653a3\",\"top\":679,\"type\":\"panelChild\",\"version\":\"2019b\",\"width\":112,\"zIndex\":1500016}"  LabelPosition=Hide
  panelInfo : PanelWebBlock  Tag=HiddenForWebPanel  PanelInfo="{\"compacted\":false,\"height\":765,\"isActiveTab\":true,\"labels\":{\"label0059391685\":{\"deleted\":false,\"left\":159,\"settings\":{\"backgroundColor\":\"rgba(0, 0, 0, 0)\",\"bold\":false,\"font\":\"Arial\",\"fontColor\":\"black\",\"fontSize\":0.9,\"italicized\":false,\"underlined\":false},\"text\":\"Presión\",\"top\":266},\"label0945694776\":{\"deleted\":false,\"left\":73,\"settings\":{\"backgroundColor\":\"rgba(0, 0, 0, 0)\",\"bold\":false,\"font\":\"Arial\",\"fontColor\":\"black\",\"fontSize\":0.9,\"italicized\":false,\"underlined\":false},\"text\":\"Actuador 3\",\"top\":733},\"label1859824746\":{\"deleted\":false,\"left\":10,\"settings\":{\"backgroundColor\":\"rgba(0, 0, 0, 0)\",\"bold\":false,\"font\":\"Arial\",\"fontColor\":\"black\",\"fontSize\":1,\"italicized\":false,\"underlined\":false},\"text\":\"ESTACIONARIA\",\"top\":208},\"label1864812803\":{\"deleted\":false,\"left\":153,\"settings\":{\"backgroundColor\":\"rgba(0, 0, 0, 0)\",\"bold\":false,\"font\":\"Arial\",\"fontColor\":\"black\",\"fontSize\":0.9,\"italicized\":false,\"underlined\":false},\"text\":\"Curvatura\",\"top\":317},\"label2804415742\":{\"deleted\":false,\"left\":252,\"settings\":{\"backgroundColor\":\"rgba(0, 0, 0, 0)\",\"bold\":false,\"font\":\"Arial\",\"fontColor\":\"black\",\"fontSize\":1,\"italicized\":false,\"underlined\":false},\"text\":\"EQUILIBRIO\",\"top\":207},\"label3298603431\":{\"deleted\":false,\"left\":67,\"settings\":{\"backgroundColor\":\"rgba(0, 0, 0, 0)\",\"bold\":true,\"font\":\"Arial\",\"fontColor\":\"black\",\"fontSize\":1,\"italicized\":false,\"underlined\":false},\"text\":\"ACTUADORES POSICIONADOS\",\"top\":343},\"label3737562089\":{\"deleted\":false,\"left\":136,\"settings\":{\"backgroundColor\":\"rgba(0, 0, 0, 0)\",\"bold\":false,\"font\":\"Arial\",\"fontColor\":\"black\",\"fontSize\":1,\"italicized\":false,\"underlined\":false},\"text\":\"DERIVATIVA\",\"top\":207},\"label4898609532\":{\"deleted\":false,\"left\":240,\"settings\":{\"backgroundColor\":\"rgba(0, 0, 0, 0)\",\"bold\":false,\"font\":\"Arial\",\"fontColor\":\"black\",\"fontSize\":0.9,\"italicized\":false,\"underlined\":false},\"text\":\"Actuador 4\",\"top\":733},\"label7245815295\":{\"deleted\":false,\"left\":68,\"settings\":{\"backgroundColor\":\"rgba(0, 0, 0, 0)\",\"bold\":false,\"font\":\"Arial\",\"fontColor\":\"black\",\"fontSize\":0.9,\"italicized\":false,\"underlined\":false},\"text\":\"Actuador 1\",\"top\":538},\"label7291504536\":{\"deleted\":false,\"left\":86,\"settings\":{\"backgroundColor\":\"rgba(0, 0, 0, 0)\",\"bold\":true,\"font\":\"Arial\",\"fontColor\":\"black\",\"fontSize\":1.1,\"italicized\":false,\"underlined\":false},\"text\":\"CONTROL AUTÓNOMO\",\"top\":22},\"label8509878005\":{\"deleted\":false,\"left\":40,\"settings\":{\"backgroundColor\":\"rgba(0, 0, 0, 0)\",\"bold\":false,\"font\":\"Arial\",\"fontColor\":\"black\",\"fontSize\":0.9,\"italicized\":false,\"underlined\":false},\"text\":\"Curvatura\",\"top\":318},\"label8762873551\":{\"deleted\":false,\"left\":127,\"settings\":{\"backgroundColor\":\"rgba(0, 0, 0, 0)\",\"bold\":true,\"font\":\"Arial\",\"fontColor\":\"black\",\"fontSize\":1,\"italicized\":false,\"underlined\":false},\"text\":\"TOLERANCIAS\",\"top\":182},\"label9049248384\":{\"deleted\":false,\"left\":234,\"settings\":{\"backgroundColor\":\"rgba(0, 0, 0, 0)\",\"bold\":false,\"font\":\"Arial\",\"fontColor\":\"black\",\"fontSize\":0.9,\"italicized\":false,\"underlined\":false},\"text\":\"Actuador 2\",\"top\":539},\"label9627187395\":{\"deleted\":false,\"left\":44,\"settings\":{\"backgroundColor\":\"rgba(0, 0, 0, 0)\",\"bold\":false,\"font\":\"Arial\",\"fontColor\":\"black\",\"fontSize\":0.9,\"italicized\":false,\"underlined\":false},\"text\":\"Presión\",\"top\":261}},\"left\":854,\"name\":\"Control Autonomo\",\"panelId\":\"panelId-e9df1c98-1b0a-4be2-b494-28bc6a7653a3\",\"tabIndex\":1,\"tabbedSetId\":\"tabbedSet0009314149\",\"top\":26,\"type\":\"panel\",\"version\":\"2019b\",\"visible\":true,\"width\":363,\"zIndex\":1500016}"  PanelSnapshot=<binary blob, 143508 chars, not shown>

== system ControlSystem_Refactorization/untitledPanel5 ==
  Linear Gauge : LinearGaugeBlock  Tag=HiddenForWebPanel  PanelInfo="{\"height\":77,\"left\":19,\"panelId\":\"panelId-ae3d63c8-6bf8-4a55-b90c-3b5066f72dcb\",\"top\":73,\"type\":\"panelChild\",\"version\":\"2019b\",\"width\":351,\"zIndex\":1500002}"  LabelPosition=Hide  ScaleMax=1  TickInterval=0.1  FontColor=[0.0, 0.0, 0.0]
  Linear Gauge1 : LinearGaugeBlock  Tag=HiddenForWebPanel  PanelInfo="{\"height\":81,\"left\":18,\"panelId\":\"panelId-ae3d63c8-6bf8-4a55-b90c-3b5066f72dcb\",\"top\":227,\"type\":\"panelChild\",\"version\":\"2019b\",\"width\":352,\"zIndex\":1500004}"  LabelPosition=Hide  ScaleMax=0.024  TickInterval=0.004  FontColor=[0.0, 0.0, 0.0]
  Linear Gauge2 : LinearGaugeBlock  Tag=HiddenForWebPanel  PanelInfo="{\"height\":91,\"left\":19,\"panelId\":\"panelId-ae3d63c8-6bf8-4a55-b90c-3b5066f72dcb\",\"top\":355,\"type\":\"panelChild\",\"version\":\"2019b\",\"width\":350,\"zIndex\":1500006}"  LabelPosition=Hide  ScaleMax=0.024  TickInterval=0.004  FontColor=[0.0, 0.0, 0.0]
  Linear Gauge3 : LinearGaugeBlock  Tag=HiddenForWebPanel  PanelInfo="{\"height\":83,\"left\":16,\"panelId\":\"panelId-ae3d63c8-6bf8-4a55-b90c-3b5066f72dcb\",\"top\":491,\"type\":\"panelChild\",\"version\":\"2019b\",\"width\":351,\"zIndex\":1500008}"  LabelPosition=Hide  ScaleMax=0.024  TickInterval=0.004  FontColor=[0.0, 0.0, 0.0]
  Linear Gauge4 : LinearGaugeBlock  Tag=HiddenForWebPanel  PanelInfo="{\"height\":85,\"left\":20,\"panelId\":\"panelId-ae3d63c8-6bf8-4a55-b90c-3b5066f72dcb\",\"top\":627,\"type\":\"panelChild\",\"version\":\"2019b\",\"width\":352,\"zIndex\":1500010}"  LabelPosition=Hide  ScaleMax=0.024  TickInterval=0.004  FontColor=[0.0, 0.0, 0.0]
  panelInfo : PanelWebBlock  Tag=HiddenForWebPanel  PanelInfo="{\"compacted\":false,\"height\":769,\"isActiveTab\":false,\"labels\":{\"label2383524707\":{\"deleted\":false,\"left\":406,\"settings\":{\"backgroundColor\":\"rgba(0, 0, 0, 0)\",\"bold\":true,\"font\":\"Arial\",\"fontColor\":\"black\",\"fontSize\":1,\"italicized\":false,\"underlined\":false},\"text\":\"E. ESTACIONARIO\",\"top\":202},\"label3335633058\":{\"deleted\":false,\"id\":\"label3335633058\",\"left\":43,\"settings\":{\"backgroundColor\":\"rgba(0, 0, 0, 0)\",\"bold\":true,\"font\":\"Arial\",\"fontColor\":\"black\",\"fontSize\":1.1,\"italicized\":false,\"underlined\":false},\"text\":\"REALIMENTACIÓN DEL REGULADOR\",\"top\":17},\"label3533013191\":{\"deleted\":false,\"id\":\"label3533013191\",\"left\":60,\"settings\":{\"backgroundColor\":\"rgba(0, 0, 0, 0)\",\"bold\":true,\"font\":\"Arial\",\"fontColor\":\"black\",\"fontSize\":1.1,\"italicized\":false,\"underlined\":false},\"text\":\"REALIMENTACIÓN DE CONTROL\",\"top\":176},\"label4096542576\":{\"deleted\":false,\"id\":\"label4096542576\",\"left\":164,\"settings\":{\"backgroundColor\":\"rgba(0, 0, 0, 0)\",\"bold\":false,\"font\":\"Arial\",\"fontColor\":\"black\",\"fontSize\":0.9,\"italicized\":false,\"underlined\":false},\"text\":\"Actuador 4\",\"top\":719},\"label4676739098\":{\"deleted\":false,\"id\":\"label4676739098\",\"left\":162,\"settings\":{\"backgroundColor\":\"rgba(0, 0, 0, 0)\",\"bold\":false,\"font\":\"Arial\",\"fontColor\":\"black\",\"fontSize\":0.9,\"italicized\":false,\"underlined\":false},\"text\":\"Actuador 1\",\"top\":311},\"label5210212135\":{\"deleted\":false,\"id\":\"label5210212135\",\"left\":146,\"settings\":{\"backgroundColor\":\"rgba(0, 0, 0, 0)\",\"bold\":true,\"font\":\"Arial\",\"fontColor\":\"black\",\"fontSize\":1,\"italicized\":false,\"underlined\":false},\"text\":\"CURVATURA\",\"top\":199},\"label5586903605\":{\"deleted\":false,\"id\":\"label5586903605\",\"left\":165,\"settings\":{\"backgroundColor\":\"rgba(0, 0, 0, 0)\",\"bold\":false,\"font\":\"Arial\",\"fontColor\":\"black\",\"fontSize\":0.9,\"italicized\":false,\"underlined\":false},\"text\":\"Actuador 3\",\"top\":581},\"label7675294442\":{\"deleted\":false,\"id\":\"label7675294442\",\"left\":160,\"settings\":{\"backgroundColor\":\"rgba(0, 0, 0, 0)\",\"bold\":true,\"font\":\"Arial\",\"fontColor\":\"black\",\"fontSize\":1,\"italicized\":false,\"underlined\":false},\"text\":\"PRESIÓN\",\"top\":39},\"label9510658439\":{\"deleted\":false,\"id\":\"label9510658439\",\"left\":161,\"settings\":{\"backgroundColor\":\"rgba(0, 0, 0, 0)\",\"bold\":false,\"font\":\"Arial\",\"fontColor\":\"black\",\"fontSize\":0.9,\"italicized\":false,\"underlined\":false},\"text\":\"Actuador 2\",\"top\":453}},\"left\":455,\"name\":\"Realimentación - Curvatura\",\"panelId\":\"panelId-ae3d63c8-6bf8-4a55-b90c-3b5066f72dcb\",\"tabIndex\":1,\"tabbedSetId\":\"tabbedSet0999669587\",\"top\":25,\"type\":\"panel\",\"version\":\"2019b\",\"visible\":false,\"width\":397,\"zIndex\":1500018}"  PanelSnapshot=<binary blob, 69544 chars, not shown>
